simulink model "FG_RealTime_EP_P2"  (R2017b)
settings: Solver=FixedStepDiscrete  StartTime=0.0  StopTime=inf  FixedStep=UserParams.SampleTime  RelTol=1e-3  EnableMultiTasking=on
InitFcn:
  | isSim = 0;
  | PreFunctions.CustomInitFcn;
model workspace (MATLAB code in the model file + MAT data in the model file):
  isSim = 0
  A_lpf_velocity_IMU = 0.0790363191017
  A_lpf_velocity_joint = 0.0790363191017
  B1_lpf_velocity_IMU = -1.56224419787
  B1_lpf_velocity_joint = -1.56224419787
  B2_lpf_velocity_IMU = 0.641280516968
  B2_lpf_velocity_joint = 0.641280516968
  Data : struct (value not decoded)
  UserParams : struct (value not decoded)
  c_CP_StanceAbdu = [0 70 40 60 0]
  c_CP_StanceKnee = [60 280 -40 -20 20]
  c_CP_SwingAbdu = [-5 -8 10 15 -5]
  c_CP_SwingKnee = [0 0 0 0 0]
  c_Gamma_st_abu = 120
  c_Gamma_st_hip = 0.5
  c_Gamma_st_knee = 150
  c_Gamma_sw_abu = 120
  c_Gamma_sw_hip = 0.1
  c_Gamma_sw_knee = 1.5
  c_Kd_abduction = 10
  c_Kd_abduction_stand = 4
  c_Kd_knee = 15
  c_Kd_knee_stand = 20
  c_Kd_lateral_stand = 0.025
  c_Kd_pitch = 40
  c_Kd_roll = 30
  c_Kd_rotation = 10
  c_Kd_rotation_stand = 4
  c_Kd_thigh = 15
  c_Kd_thigh_stand = 10
  c_Kd_toe = 2
  c_Kd_toe_stand = 80
  c_Kd_yaw = 4
  c_Kfl_d = 0.5
  c_Kfl_p = 0.25
  c_Kfs_d = 0.08
  c_Kfs_p = 0.05
  c_Kp_abduction = 600
  c_Kp_abduction_stand = 400
  c_Kp_knee = 500
  c_Kp_knee_stand = 500
  c_Kp_lateral_stand = 2
  c_Kp_pitch = 800
  c_Kp_roll = 500
  c_Kp_rotation = 800
  c_Kp_rotation_stand = 200
  c_Kp_thigh = 500
  c_Kp_thigh_stand = 200
  c_Kp_toe = 10
  c_Kp_toe_stand = 600
  c_Kp_yaw = 200
  c_abduction_inward_gain = 1
  c_com_bp = 0.05
  c_fil_para_2 = 0.02
  c_fil_para_3 = 0.02
  c_fil_para_4 = 0.001
  c_fil_para_5 = 0.02
  c_fil_para_x = 0.002
  c_fil_para_y = 0.002
  c_fil_vel_offset = 0
  c_final_st_abduction = 0.05
  c_final_sw_abduction = 0.15
  c_force_step_end_s = 1
  c_init_lateral_velocity = 0.1
  c_joint_filter_choice = 1
  c_lateral_offset_exp = 0
  c_lateral_velocity_weight = 1
  c_pre_final_sw_abduction = -0.01
  c_sagittal_offset_exp = 0
  c_sagittal_speed = 0
  c_shift_distance = 0.03
  c_shift_time = 0.4
  c_stance_thre_lb = 100
  c_stance_thre_ub = 200
  c_stand_offset_exp = 0
  c_standing_switch_time = 0.4
  c_toe_tilt_angle = 0
  c_turning_offset_exp = 0
  c_u_abduction_cp = 40
  c_u_abduction_swing_cp = 14
  c_u_knee_cp = 120
  c_u_thigh_cp = -15
  cassieDataBusInfo : struct (value not decoded)
  fcut_velocity_IMU = 628.318530718
  fcut_velocity_joint = 628.318530718
  lpf_damping = 0.707106781187
  sample_time = 0.0005
  other statements: CassieModule.importBuses;; PreFunctions.CustomInitFcn;
symbols that are objects in the model workspace (value not decoded): UserParams
undefined symbols (not defined in the file or in its folder): BusModule, getMocapDataStruct, getSlrtDataStruct
libraries: slrtlib x116, xpcrtudplib x2, CassieLibrary x1, simulink x1, func_block_library x1
(part 3 of 3)

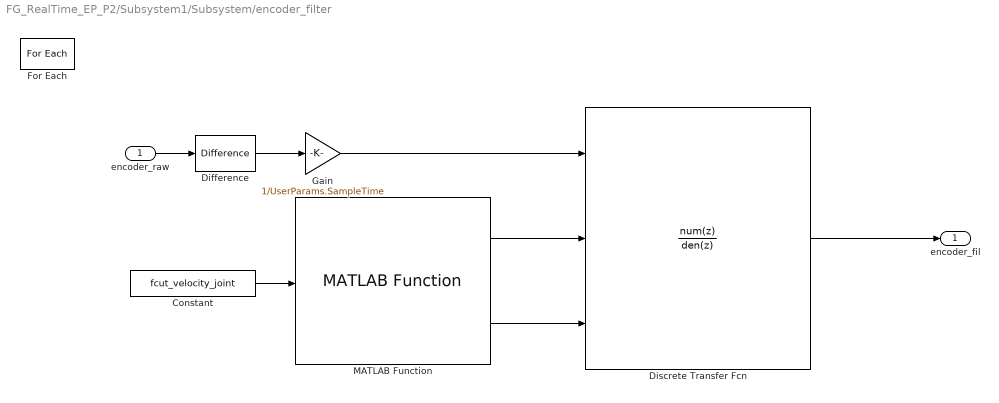
== system FG_RealTime_EP_P2/Subsystem1/Subsystem/encoder_filter ==
  encoder_raw : Inport  Partition=on  PartitionDimension=1  PartitionWidth=1  PartitionOffset=0
  Constant : Constant  Value=fcut_velocity_joint
  Difference : simulink/Discrete/Difference  ICPrevInput=0.0  OutMin=[]  OutMax=[]  OutDataType=fixdt(1, 16)  OutScaling=2^-10  DoSatur=off
  Discrete Transfer Fcn : DiscreteTransferFcn  NumeratorSource=Input port  DenominatorSource=Input port  SampleTime=UserParams.SampleTime  a0EqualsOne=on
      settings: InputPortMap=u0,p1,p3
  For Each : ForEach  DisableCoverage=on  IndexMode=One-based
  Gain : Gain  Gain=1/UserParams.SampleTime
  MATLAB Function : func_block_library/MATLAB Function
  encoder_fil : Outport  ConcatenationDimension=1
  wires:
  MATLAB Function/2 -> Discrete Transfer Fcn/3
  MATLAB Function/1 -> Discrete Transfer Fcn/2
  Discrete Transfer Fcn/1 -> encoder_fil/1
  Gain/1 -> Discrete Transfer Fcn/1
  Difference/1 -> Gain/1
  Constant/1 -> MATLAB Function/1
  encoder_raw/1 -> Difference/1
